simulink model "secondOrderComplFilter"  (R2019a)
settings: Solver=VariableStepAuto  StartTime=0.0  StopTime=30  RelTol=1e-3
values from neighbouring files (symbols this model uses):
  T = 0.6    [secondOrderComplFilter_param.m]
undefined symbols (not defined in the file or in its folder): DiscIntNeverNeededParam
libraries: eeGeneralControl x3
settings Model: Creator=christinefux  LastModifiedBy=christinefux

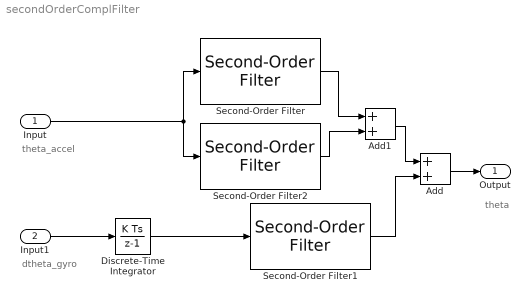
== system secondOrderComplFilter ==
  note: theta
  note: dtheta_gyro
  note: theta_accel
  Input : Inport
  Input1 : Inport  Port=2
  Add : Sum
  Add1 : Sum
  Discrete-Time Integrator : DiscreteIntegrator  SampleTime=-1  ICPrevOutput=DiscIntNeverNeededParam  ICPrevScaledInput=DiscIntNeverNeededParam
  Second-Order Filter : eeGeneralControl/Second-Order Filter  FilterType=Low-pass  fn=2*pi/T  Zeta=d  Ts=0  A0=0  Ph0=0  f0=0  b0=0
      settings: SourceProductName=Simscape Electrical  SourceProductBaseCode=PS
  Second-Order Filter1 : eeGeneralControl/Second-Order Filter  FilterType=High-pass  fn=2*pi/T  Zeta=d  Ts=0  A0=0  Ph0=0  f0=0  b0=0
      settings: SourceProductName=Simscape Electrical  SourceProductBaseCode=PS
  Second-Order Filter2 : eeGeneralControl/Second-Order Filter  FilterType=Band-pass  fn=2*pi/T  Zeta=d  Ts=0  A0=0  Ph0=0  f0=0  b0=0
      settings: SourceProductName=Simscape Electrical  SourceProductBaseCode=PS
  Output : Outport
  wires:
  Input1/1 -> Discrete-Time Integrator/1
  Second-Order Filter1/1 -> Add/2
  Add/1 -> Output/1
  Second-Order Filter/1 -> Add1/1
  Second-Order Filter2/1 -> Add1/2
  Add1/1 -> Add/1
  Input/1 -> Second-Order Filter/1, Second-Order Filter2/1
  Discrete-Time Integrator/1 -> Second-Order Filter1/1
